simulink model "psk8"  (R2020a)
settings: Solver=VariableStepAuto  StartTime=0.0  StopTime=10.0  RelTol=1e-3
libraries: commdigbbndpm3 x2, commchan3 x1, commrandsrc3 x1
settings Model: Creator=uzend  LastModifiedBy=uzend

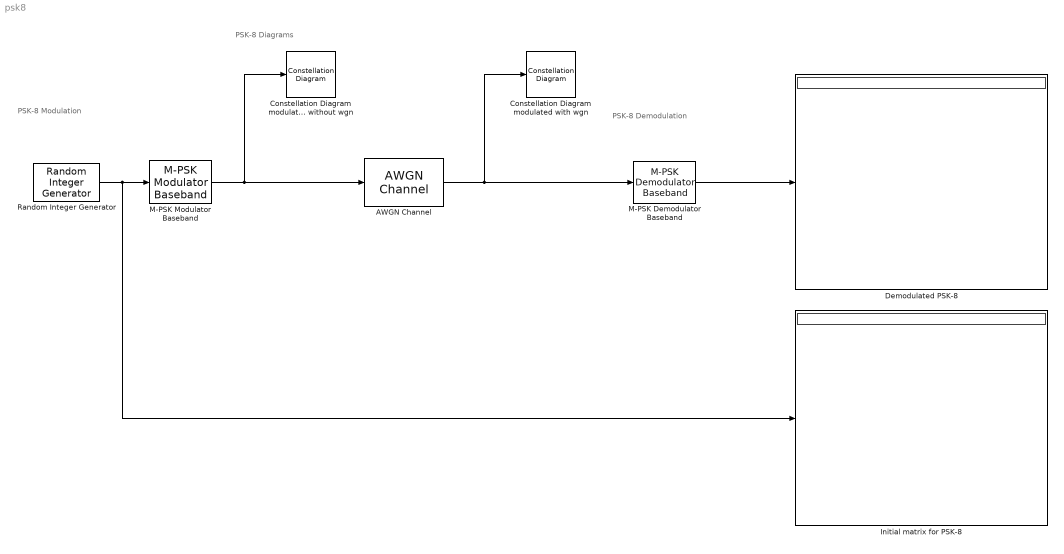
== system psk8 ==
  note: PSK-8 Demodulation
  note: PSK-8 Diagrams
  note: PSK-8 Modulation
  AWGN Channel : commchan3/AWGN Channel  InputProcessing=Columns as channels (frame based)  seed=67  noiseMode="Signal to noise ratio  (Eb/No)"  EbNodB=25  EsNodB=10  SNRdB=10  bitsPerSym=1  Ps=1  Tsym=1  variance=1
  Constellation Diagram modulated with wgn : ConstellationDiagram
  Constellation Diagram modulated without wgn : ConstellationDiagram
  Demodulated PSK-8 : Display
  Initial matrix for PSK-8 : Display
  M-PSK Demodulator Baseband : commdigbbndpm3/M-PSK Demodulator Baseband  M=8  OutType=Integer  DecType=Hard decision  VarSource=Dialog  Variance=1  Dec=User-defined  Mapping=[0:7]  Ph=pi/8  outDtype1=Inherit via internal rule  outDtype2=Inherit via internal rule  derotateFactorWordLen=16  derotateFactorDataTypeStr=Inherit: Same word length as input  derotateFactorLastDataTypeStr=Inherit: Same word length as input
  M-PSK Modulator Baseband : commdigbbndpm3/M-PSK Modulator Baseband  M=8  InType=Integer  Enc=User-defined  Mapping=[0:7]  Ph=pi/8  outDtype=double  outWordLen=16  outUDDataType=sfix(16)  outFracLenMode=Best precision  outFracLen=15  outDataTypeStr=double  outLastDataTypeStr=double
  Random Integer Generator : commrandsrc3/Random Integer Generator  SetSize=8  SeedSource=Auto  Seed=0  SampleTime=1  SamplesPerFrame=100  OutputDataType=double  SimulateUsing=Interpreted execution
  wires:
  M-PSK Modulator Baseband/1 -> AWGN Channel/1, Constellation Diagram modulated without wgn/1
  AWGN Channel/1 -> M-PSK Demodulator Baseband/1, Constellation Diagram modulated with wgn/1
  Random Integer Generator/1 -> M-PSK Modulator Baseband/1, Initial matrix for PSK-8/1
  M-PSK Demodulator Baseband/1 -> Demodulated PSK-8/1
